simulink model "joint_test_dis_massless_2GBlks1"  (R2013a)
settings: Solver=ode45  StartTime=0.0  StopTime=10.0  RelTol=1e-3
libraries: sm_lib x7
settings Model: Creator=smiller  LastModifiedBy=smiller

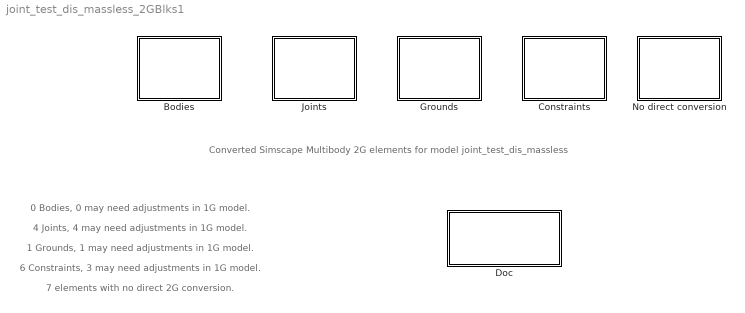
== system joint_test_dis_massless_2GBlks1 ==
  note: Converted Simscape Multibody 2G elements for model
      | joint_test_dis_massless
  note: 0 Bodies, 0 may need adjustments in 1G model.
  note: 4 Joints, 4 may need adjustments in 1G model.
  note: 1 Grounds, 1 may need adjustments in 1G model.
  note: 6 Constraints, 3 may need adjustments in 1G model.
  note: 7 elements with no direct 2G conversion.
  Bodies : Subsystem
  Constraints : Subsystem
  Doc : Subsystem
      settings: OpenFcn=web('SM1G2G_Warnings_Help.html');
      mask Display: disp('Double-click\nfor Information\nabout Diagnostics');
  Grounds : Subsystem
  Joints : Subsystem
  No direct conversion : Subsystem

== system joint_test_dis_massless_2GBlks1/Bodies ==

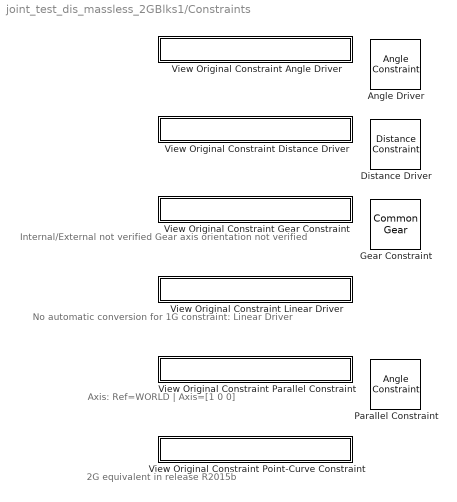
== system joint_test_dis_massless_2GBlks1/Constraints ==
  note: Internal/External not verified
      | Gear axis orientation not verified
  note: No automatic conversion for 1G constraint: Linear Driver
  note: Axis: Ref=WORLD | Axis=[1 0 0]
  note: 2G equivalent in release R2015b
  Angle Driver : sm_lib/Constraints/Angle  Constraint  ConstraintType=General  Angle=0  AngleUnits=deg  SenseTorque=off  BlockFunction=simmechanics.library.constraints.angle_constraint
  Distance Driver : sm_lib/Constraints/Distance  Constraint  Distance=0  DistanceUnits=m  SenseForce=off  BlockFunction=simmechanics.library.constraints.distance_constraint
  Gear Constraint : sm_lib/Gears, Couplings and Drives/Gears/Common Gear  GearType=External  SpecificationType=PitchCircleRadii  CenterDistance=20.0  CenterDistanceUnits=cm  GearRatio=1.0  BaseGearRadius=1  BaseGearRadiusUnits=m  FollGearRadius=1  FollGearRadiusUnits=m  AssemblyGearRotation=Free  BlockFunction=simmechanics.library.gears_couplings_drives.gears.common_gear
  Parallel Constraint : sm_lib/Constraints/Angle  Constraint  ConstraintType=Parallel  Angle=0  AngleUnits=deg  SenseTorque=off  BlockFunction=simmechanics.library.constraints.angle_constraint
  View Original Constraint Angle Driver : Subsystem
      settings: OpenFcn=hilite_system('joint_test_dis_massless/Angle Driver');
      mask Display: disp(['View Original Constraint Angle Driver']);
  View Original Constraint Distance Driver : Subsystem
      settings: OpenFcn=hilite_system('joint_test_dis_massless/Distance Driver');
      mask Display: disp(['View Original Constraint Distance Driver']);
  View Original Constraint Gear Constraint : Subsystem
      settings: OpenFcn=hilite_system('joint_test_dis_massless/Gear Constraint');
      mask Display: disp(['View Original Constraint Gear Constraint']);
  View Original Constraint Linear Driver : Subsystem
      settings: OpenFcn=hilite_system('joint_test_dis_massless/Linear Driver');
      mask Display: disp(['View Original Constraint Linear Driver']);
  View Original Constraint Parallel Constraint : Subsystem
      settings: OpenFcn=hilite_system('joint_test_dis_massless/Parallel Constraint');
      mask Display: disp(['View Original Constraint Parallel Constraint']);
  View Original Constraint Point-Curve Constraint : Subsystem
      settings: OpenFcn=hilite_system('joint_test_dis_massless/Point-Curve Constraint');
      mask Display: disp(['View Original Constraint Point-Curve Constraint']);

== system joint_test_dis_massless_2GBlks1/Doc ==

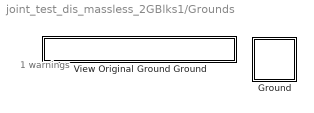
== system joint_test_dis_massless_2GBlks1/Grounds ==
  note: 1 warnings
  Ground : Subsystem
  View Original Ground Ground : Subsystem
      settings: OpenFcn=hilite_system('joint_test_dis_massless/Ground');
      mask Display: disp(['View Original Ground Ground']);

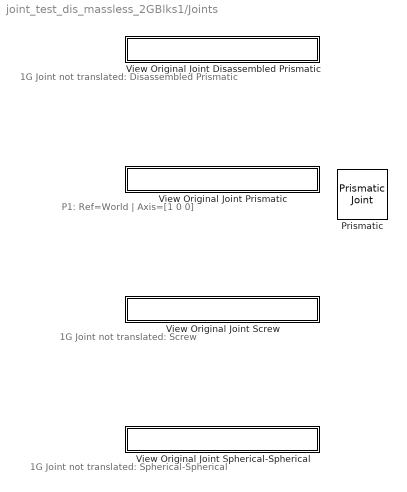
== system joint_test_dis_massless_2GBlks1/Joints ==
  note: 1G Joint not translated: Disassembled Prismatic
  note: P1: Ref=World | Axis=[1 0 0]
  note: 1G Joint not translated: Screw
  note: 1G Joint not translated: Spherical-Spherical
  Prismatic : sm_lib/Joints/Prismatic  Joint  SenseConstraintForceX=off  SenseConstraintForceY=off  SenseConstraintForceZ=off  SenseConstraintTorqueX=off  SenseConstraintTorqueY=off  SenseConstraintTorqueZ=off  ConstraintWrenchDir=FollowerOnBase  ConstraintWrenchFrame=BaseFrame  EquilibriumPosition=0  EquilibriumPositionUnits=m  SpringStiffness=0  SpringStiffnessUnits=N/m  DampingCoefficient=0  DampingCoefficientUnits=N/(m/s)  ActuationMode=NoActuation  SensePosition=off  SenseVelocity=off  SenseAcceleration=off  SenseTorqueForce=off  PositionTargetValue=0  PositionTargetValueUnits=m  PositionTargetSpecify=off  PositionTargetPriority=High  VelocityTargetValue=0  VelocityTargetValueUnits=m/s  VelocityTargetSpecify=off  VelocityTargetPriority=High  BlockFunction=simmechanics.library.joints.prismatic_joint
  View Original Joint Disassembled Prismatic : Subsystem
      settings: OpenFcn=hilite_system('joint_test_dis_massless/Disassembled Prismatic');
      mask Display: disp([' View Original Joint Disassembled Prismatic']);
  View Original Joint Prismatic : Subsystem
      settings: OpenFcn=hilite_system('joint_test_dis_massless/Prismatic');
      mask Display: disp([' View Original Joint Prismatic']);
  View Original Joint Screw : Subsystem
      settings: OpenFcn=hilite_system('joint_test_dis_massless/Screw');
      mask Display: disp([' View Original Joint Screw']);
  View Original Joint Spherical-Spherical : Subsystem
      settings: OpenFcn=hilite_system('joint_test_dis_massless/Spherical-Spherical');
      mask Display: disp([' View Original Joint Spherical-Spherical']);

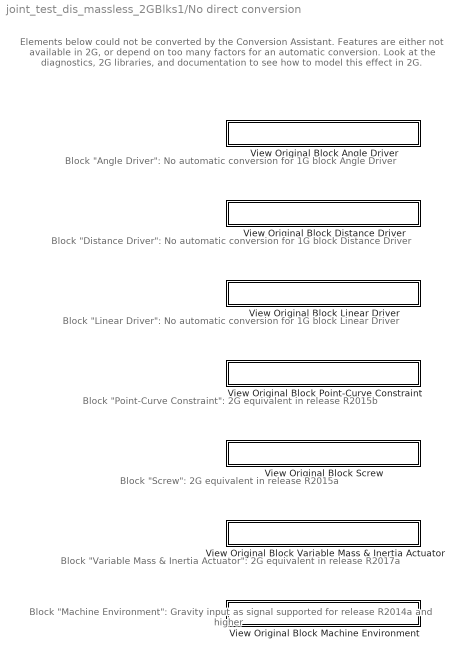
== system joint_test_dis_massless_2GBlks1/No direct conversion ==
  note: Block "Angle Driver": No automatic conversion for 1G block Angle Driver
  note: Block "Distance Driver": No automatic conversion for 1G block Distance Driver
  note: Block "Linear Driver": No automatic conversion for 1G block Linear Driver
  note: Block "Point-Curve Constraint": 2G equivalent in release R2015b
  note: Block "Screw": 2G equivalent in release R2015a
  note: Block "Variable Mass & Inertia Actuator": 2G equivalent in release R2017a
  note: Block "Machine Environment": Gravity input as signal supported for release R2014a and higher
  note: Elements below could not be converted by the Conversion Assistant.
      | Features are either not available in 2G, or depend on too many factors
      | for an automatic conversion. Look at the diagnostics, 2G libraries, and
      | documentation to see how to model this effect in 2G.
  View Original Block Angle Driver : Subsystem
      settings: OpenFcn=hilite_system('joint_test_dis_massless/Angle Driver');
      mask Display: disp([' View Original Block Angle Driver']);
  View Original Block Distance Driver : Subsystem
      settings: OpenFcn=hilite_system('joint_test_dis_massless/Distance Driver');
      mask Display: disp([' View Original Block Distance Driver']);
  View Original Block Linear Driver : Subsystem
      settings: OpenFcn=hilite_system('joint_test_dis_massless/Linear Driver');
      mask Display: disp([' View Original Block Linear Driver']);
  View Original Block Machine Environment : Subsystem
      settings: OpenFcn=hilite_system('joint_test_dis_massless/Machine Environment');
      mask Display: disp([' View Original Block Machine Environment']);
  View Original Block Point-Curve Constraint : Subsystem
      settings: OpenFcn=hilite_system('joint_test_dis_massless/Point-Curve Constraint');
      mask Display: disp([' View Original Block Point-Curve Constraint']);
  View Original Block Screw : Subsystem
      settings: OpenFcn=hilite_system('joint_test_dis_massless/Screw');
      mask Display: disp([' View Original Block Screw']);
  View Original Block Variable Mass & Inertia Actuator : Subsystem
      settings: OpenFcn=hilite_system('joint_test_dis_massless/Variable Mass & Inertia Actuator');
      mask Display: disp([' View Original Block Variable Mass & Inertia Actuator']);

== system joint_test_dis_massless_2GBlks1/Constraints/View Original Constraint Angle Driver ==

== system joint_test_dis_massless_2GBlks1/Constraints/View Original Constraint Distance Driver ==

== system joint_test_dis_massless_2GBlks1/Constraints/View Original Constraint Gear Constraint ==

== system joint_test_dis_massless_2GBlks1/Constraints/View Original Constraint Linear Driver ==

== system joint_test_dis_massless_2GBlks1/Constraints/View Original Constraint Parallel Constraint ==

== system joint_test_dis_massless_2GBlks1/Constraints/View Original Constraint Point-Curve Constraint ==

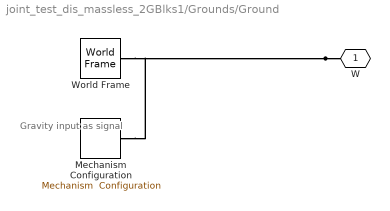
== system joint_test_dis_massless_2GBlks1/Grounds/Ground ==
  note: Gravity input as signal
  Mechanism Configuration : sm_lib/Utilities/Mechanism  Configuration  GravityVector=[0 -9.81 0]  GravityUnits=m/s^2  AllowGravitySignal=off  LinearizationDelta=0.001  BlockFunction=simmechanics.library.utilities.mechanism_configuration
  World Frame : sm_lib/Frames and  Transforms/World Frame  BlockFunction=simmechanics.library.frames_transforms.world_frame
  W : PMIOPort  Port=1  Side=Right
  connections:
  W/RConn1 -- World Frame/RConn1 -- Mechanism Configuration/RConn1

== system joint_test_dis_massless_2GBlks1/Grounds/View Original Ground Ground ==

== system joint_test_dis_massless_2GBlks1/Joints/View Original Joint Disassembled Prismatic ==

== system joint_test_dis_massless_2GBlks1/Joints/View Original Joint Prismatic ==

== system joint_test_dis_massless_2GBlks1/Joints/View Original Joint Screw ==

== system joint_test_dis_massless_2GBlks1/Joints/View Original Joint Spherical-Spherical ==

== system joint_test_dis_massless_2GBlks1/No direct conversion/View Original Block Angle Driver ==

== system joint_test_dis_massless_2GBlks1/No direct conversion/View Original Block Distance Driver ==

== system joint_test_dis_massless_2GBlks1/No direct conversion/View Original Block Linear Driver ==

== system joint_test_dis_massless_2GBlks1/No direct conversion/View Original Block Machine Environment ==

== system joint_test_dis_massless_2GBlks1/No direct conversion/View Original Block Point-Curve Constraint ==

== system joint_test_dis_massless_2GBlks1/No direct conversion/View Original Block Screw ==

== system joint_test_dis_massless_2GBlks1/No direct conversion/View Original Block Variable Mass & Inertia Actuator ==
